simulink model "stage5_2D"  (R2025b)
settings: Solver=FixedStepDiscrete  StartTime=0.0  StopTime=stopTime  FixedStep=dt  RelTol=1e-3
undefined symbols (not defined in the file): A, B, C1, C2, dt, H, K_seq, L_seq, N, noiseOn, sdMat, seedC1, seedC2, seedS, spread, X1
settings Model: Creator=parimalsaha  LastModifiedBy=parimalsaha
settings DataIOCC: ReturnWorkspaceOutputs=off
settings DebuggingCC: AlgebraicLoopMsg=error

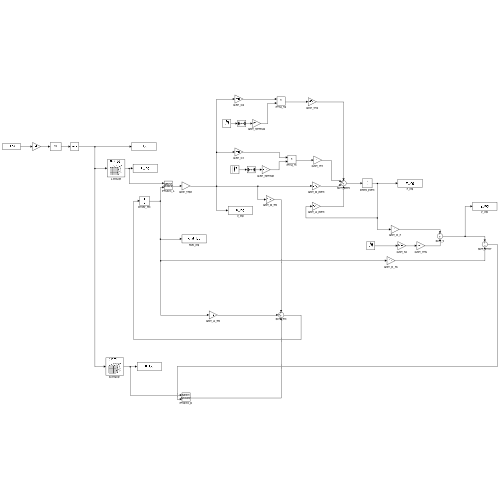
[thumbnail: Simulink's stored preview of the top-level diagram]
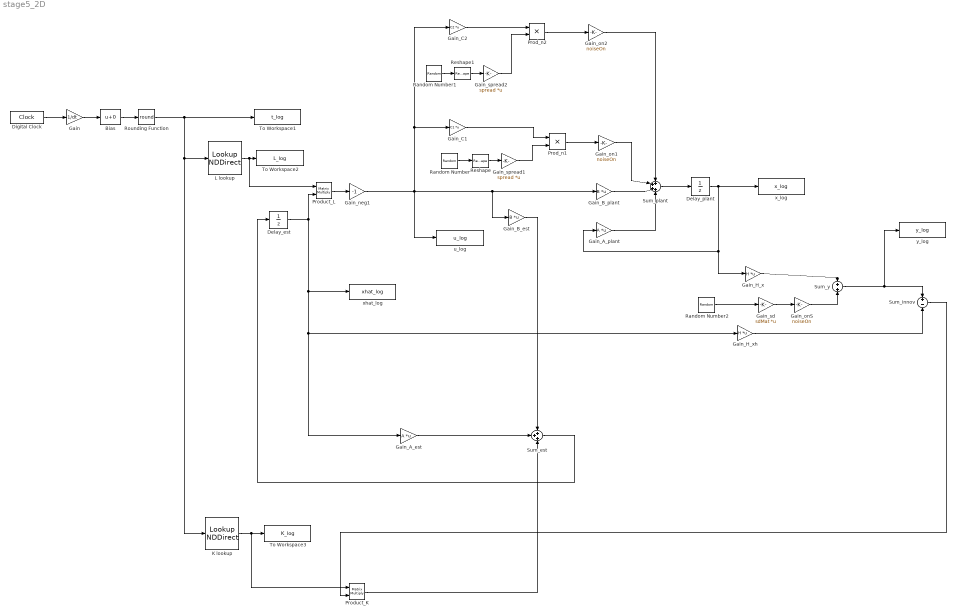
== system stage5_2D ==
  Bias : Bias  SaturateOnIntegerOverflow=off
  Delay_est : UnitDelay  InitialCondition=X1  SampleTime=dt  HasFrameUpgradeWarning=on
  Delay_plant : UnitDelay  InitialCondition=X1  SampleTime=dt  HasFrameUpgradeWarning=on
  Digital Clock : DigitalClock  SampleTime=dt
  Gain : Gain  Gain=1/dt
  Gain_A_est : Gain  Gain=A  Multiplication=Matrix(K*u)
  Gain_A_plant : Gain  Gain=A  Multiplication=Matrix(K*u)
  Gain_B_est : Gain  Gain=B  Multiplication=Matrix(K*u)
  Gain_B_plant : Gain  Gain=B  Multiplication=Matrix(K*u)
  Gain_C1 : Gain  Gain=C1  Multiplication=Matrix(K*u)
  Gain_C2 : Gain  Gain=C2  Multiplication=Matrix(K*u)
  Gain_H_x : Gain  Gain=H  Multiplication=Matrix(K*u)
  Gain_H_xh : Gain  Gain=H  Multiplication=Matrix(K*u)
  Gain_neg1 : Gain  Gain=-1
  Gain_on1 : Gain  Gain=noiseOn
  Gain_on2 : Gain  Gain=noiseOn
  Gain_onS : Gain  Gain=noiseOn
  Gain_sd : Gain  Gain=sdMat  Multiplication=Matrix(K*u)
  Gain_spread1 : Gain  Gain=spread  Multiplication=Matrix(K*u)
  Gain_spread2 : Gain  Gain=spread  Multiplication=Matrix(K*u)
  "K lookup " : LookupNDDirect  NumberOfTableDimensions=3  InputsSelectThisObjectFromTable=2-D Matrix  Table=K_seq  DiagnosticForOutOfRangeInput=Error
  L lookup : LookupNDDirect  NumberOfTableDimensions=3  InputsSelectThisObjectFromTable=2-D Matrix  Table=L_seq  DiagnosticForOutOfRangeInput=Error
  Prod_n1 : Product
  Prod_n2 : Product
  Product_K : Product  Multiplication=Matrix(*)
  Product_L : Product  Multiplication=Matrix(*)
  Random Number : RandomNumber  Seed=seedC1  SampleTime=dt
  Random Number1 : RandomNumber  Seed=seedC2  SampleTime=dt
  Random Number2 : RandomNumber  Seed=seedS  SampleTime=dt
  Reshape : Reshape  OutputDimensionality=Row vector (2-D)  OutputDimensions=[1 N]
  Reshape1 : Reshape  OutputDimensionality=Row vector (2-D)  OutputDimensions=[1 N]
  Rounding Function : Rounding  Operator=round
  Sum_est : Sum  Inputs=+++
  Sum_innov : Sum  Inputs=+-
  Sum_plant : Sum  Inputs=++++
  Sum_y : Sum
  To Workspace1 : ToWorkspace  VariableName=t_log  SampleTime=dt
  To Workspace2 : ToWorkspace  VariableName=L_log  SampleTime=-1
  To Workspace3 : ToWorkspace  VariableName=K_log  SampleTime=-1
  u_log : ToWorkspace  VariableName=u_log  SampleTime=-1
  x_log : ToWorkspace  VariableName=x_log  SampleTime=dt
  xhat_log : ToWorkspace  VariableName=xhat_log  SampleTime=-1
  y_log : ToWorkspace  VariableName=y_log  SampleTime=-1
  wires:
  Sum_plant/1 -> Delay_plant/1
  Delay_plant/1 -> Gain_H_x/1, Gain_A_plant/1, x_log/1
  Digital Clock/1 -> Gain/1
  Gain/1 -> Bias/1
  Bias/1 -> Rounding Function/1
  Rounding Function/1 -> To Workspace1/1, L lookup/1, "K lookup "/1
  L lookup/1 -> Product_L/1, To Workspace2/1
  "K lookup "/1 -> Product_K/1, To Workspace3/1
  Delay_est/1 -> xhat_log/1, Gain_H_xh/1, Gain_A_est/1, Product_L/2
  Product_L/1 -> Gain_neg1/1
  Gain_H_xh/1 -> Sum_innov/2
  Sum_innov/1 -> Product_K/2
  Gain_B_est/1 -> Sum_est/1
  Gain_A_est/1 -> Sum_est/2
  Product_K/1 -> Sum_est/3
  Sum_est/1 -> Delay_est/1
  Gain_neg1/1 -> Gain_C2/1, Gain_C1/1, u_log/1, Gain_B_plant/1, Gain_B_est/1
  Gain_C1/1 -> Prod_n1/1
  Gain_spread1/1 -> Prod_n1/2
  Prod_n1/1 -> Gain_on1/1
  Gain_A_plant/1 -> Sum_plant/4
  Gain_B_plant/1 -> Sum_plant/3
  Gain_on1/1 -> Sum_plant/2
  Gain_C2/1 -> Prod_n2/1
  Gain_spread2/1 -> Prod_n2/2
  Prod_n2/1 -> Gain_on2/1
  Gain_on2/1 -> Sum_plant/1
  Gain_H_x/1 -> Sum_y/1
  Gain_sd/1 -> Gain_onS/1
  Gain_onS/1 -> Sum_y/2
  Sum_y/1 -> y_log/1, Sum_innov/1
  Reshape/1 -> Gain_spread1/1
  Random Number/1 -> Reshape/1
  Random Number2/1 -> Gain_sd/1
  Random Number1/1 -> Reshape1/1
  Reshape1/1 -> Gain_spread2/1
